simulink model "LabB_PIDOverRobot"  (R2019b)
settings: Solver=FixedStepDiscrete  StartTime=0.0  StopTime=inf  FixedStep=fSamplingPeriod  RelTol=1e-3  EnableMultiTasking=on
values from neighbouring files (symbols this model uses):
  fGyroBias = -315    [GyroBias.mat]
  fGyroConversionFactor = -1/131    (= -0.00763358778626)    [LabB_ObserverAndControllerOverRobot_Parameters.m]    (also in LabB_PIDOverRobot_Parameters.m; LabC_Servo.m; LabC_observer.m; LoadRobotParameters.m = 0.00762939453125)
  fSamplingPeriod = 0.005    [LabB_ControllerOverSimulator_Discrete_Parameters.m]    (also in LabB_ObserverAndControllerOverRobot_Parameters.m = 0.01; LabB_ObserverAndControllerOverSimulator_Discrete_Parameters.m = 0.01; LabB_ObserverOverSimulator_Discrete_Parameters.m = 0.01; LabB_PIDOverRobot_Parameters.m)
  fWheelRadius = 0.0216    [LabB_ObserverAndControllerOverRobot_Parameters.m]    (also in LabB_PIDOverRobot_Parameters.m; LabC_Servo.m; LabC_observer.m; LoadRobotParameters.m)
  iNumberOfEncoderSteps = 720    [LabB_ObserverAndControllerOverRobot_Parameters.m]    (also in LabB_PIDOverRobot_Parameters.m; LabC_Servo.m; LabC_observer.m; LoadRobotParameters.m)
  kD = -0.0554    [LabB_ObserverAndControllerOverRobot_Parameters.m]    (also in LabB_ObserverAndControllerOverSimulator_Discrete_Parameters.m; LabB_ObserverOverSimulator_Continuous_Parameters.m = -0.0553889349754; LabB_ObserverOverSimulator_Discrete_Parameters.m = -0.0553889349754; LabB_PIDOverRobot_Parameters.m = -0.05538361401)
  kI = -263.4728    [LabB_ObserverAndControllerOverRobot_Parameters.m]    (also in LabB_ObserverAndControllerOverSimulator_Discrete_Parameters.m; LabB_ObserverOverSimulator_Continuous_Parameters.m = -263.472756557; LabB_ObserverOverSimulator_Discrete_Parameters.m = -263.472756557; LabB_PIDOverRobot_Parameters.m = -263.540867)
  kP = -47.0274    [LabB_ObserverAndControllerOverRobot_Parameters.m]    (also in LabB_ObserverAndControllerOverSimulator_Discrete_Parameters.m; LabB_ObserverOverSimulator_Continuous_Parameters.m = -47.0274213515; LabB_ObserverOverSimulator_Discrete_Parameters.m = -47.0274213515; LabB_PIDOverRobot_Parameters.m = -47.0230144)
undefined symbols (not defined in the file or in its folder): DiscIntNeverNeededParam
libraries: MinSegLibrary_M2V3 x3, simulink x1
settings Model: FPTRunName=FPA_Reference  ExtModeTrigDuration=2  Creator=Alec  LastModifiedBy=jlosi
settings DataIOCC: SaveFormat=Array  SaveOutput=off  SignalLogging=off  DSMLogging=off  SaveTime=off  ReturnWorkspaceOutputs=off
settings OptimizationCC: PassReuseOutputArgsAs=Individual arguments  ExpressionDepthLimit=2147483647  MaxStackSize=64  EfficientTunableParamExpr=on
settings DebuggingCC: UnderspecifiedInitializationDetection=Classic  MergeDetectMultiDrivingBlocksExec=none  ParameterTunabilityLossMsg=error  StateNameClashWarn=warning  SFUnexpectedBacktrackingDiag=warning  SFNoUnconditionalDefaultTransitionDiag=warning  SFExecutionAtInitializationDiag=none  ArithmeticOperatorsInVariantConditions=warning
settings HardwareCC: ProdBitPerInt=16  ProdBitPerPointer=16  ProdBitPerSizeT=16  ProdBitPerPtrDiffT=16  ProdLargestAtomicFloat=None  ProdWordSize=8  ProdHWDeviceType=Atmel->AVR
settings ModelReferenceCC: PropagateSignalLabelsOutOfModel=off
settings SFSimCC: SimUseLocalCustomCode=off  MATLABDynamicMemAlloc=off  CustomCodeUndefinedFunction=UseInterfaceOnly
settings RTWCC: SystemTargetFile=ert.tlc  HardwareBoard=Arduino Mega 2560  TLCOptions=-aInlineSetEventsForThisBaseRateFcn=TLC_FALSE -aSuppressMultiTaskScheduler=TLC_FALSE -aRateBasedStepFcn=1  TemplateMakefile=ert_default_tmf  GenerateReport=on  RTWVerbose=off  RTWUseLocalCustomCode=off  Toolchain=Arduino AVR  BuildConfiguration=Faster Runs  IncludeHyperlinkInReport=on  LaunchReport=on  GenerateTraceInfo=on  GenerateTraceReport=on  GenerateTraceReportSl=on  GenerateTraceReportSf=on  GenerateTraceReportEml=on
settings CodeAppCC: ForceParamTrailComments=on  IgnoreCustomStorageClasses=off  OperatorAnnotations=on  SimulinkDataObjDesc=on  SFDataObjDesc=on  MATLABFcnDesc=on  CustomSymbolStrType=$N$R$M  InsertBlockDesc=on  StateflowObjectComments=on  MATLABSourceComments=on  InternalIdentifier=Classic
settings ERTTargetCC: SupportContinuousTime=on  SupportVariableSizeSignals=on
settings ConfigComp: CovMetricSettings=dw  CovHtmlReporting=on  CovSaveCumulativeToWorkspaceVar=on  CovSaveSingleToWorkspaceVar=on  CovExternalEMLEnable=off

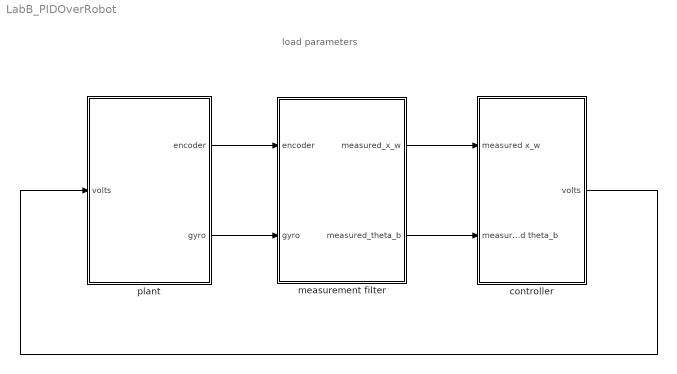
== system LabB_PIDOverRobot ==
  note: load parameters
  controller : Subsystem
  measurement filter : Subsystem
  plant : Subsystem
  wires:
  controller/1(volts) -> plant/1(volts)
  plant/2(gyro) -> measurement filter/2(gyro)
  measurement filter/2(measured_theta_b) -> controller/2("measured theta_b ")
  measurement filter/1(measured_x_w) -> controller/1(measured x_w)
  plant/1(encoder) -> measurement filter/1(encoder)

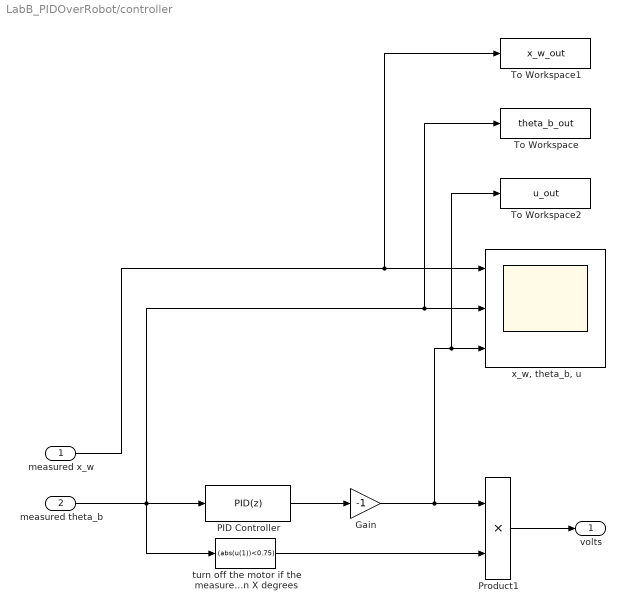
== system LabB_PIDOverRobot/controller ==
  measured x_w : Inport
  "measured theta_b " : Inport  Port=2
  Gain : Gain  Gain=-1
  PID Controller : simulink/Continuous/PID Controller  Controller=PID  Form=Parallel  TimeDomain=Discrete-time  SampleTime=fSamplingPeriod  IntegratorMethod=Forward Euler  FilterMethod=Forward Euler  ControllerParametersSource=internal  P=-kP  I=-kI  D=-kD  UseFilter=on  N=100  TunerSelectOption=Transfer Function Based (PID Tuner App)  InitialConditionSource=internal  InitialConditionForIntegrator=0  InitialConditionForFilter=0  DifferentiatorICPrevScaledInput=0  ExternalReset=none  TrackingMode=off  Kt=1  LimitOutput=on  UpperSaturationLimit=6  LowerSaturationLimit=-6  LinearizeAsGain=on  AntiWindupMode=back-calculation  Kb=1  POutMin=[]  POutMax=[]  IOutMin=[]  IOutMax=[]  DOutMin=[]  DOutMax=[]  NOutMin=[]  NOutMax=[]  SumOutMin=[]  SumOutMax=[]  SaturationOutMin=[]  SaturationOutMax=[]  PParamMin=[]  PParamMax=[]  IParamMin=[]  IParamMax=[]  DParamMin=[]  DParamMax=[]  NParamMin=[]  NParamMax=[]  KbParamMin=[]  KbParamMax=[]  KtParamMin=[]  KtParamMax=[]  KbOutMin=[]  KbOutMax=[]  KtOutMin=[]  KtOutMax=[]  IntegratorOutMin=[]  IntegratorOutMax=[]  FilterOutMin=[]  FilterOutMax=[]  SumI1OutMin=[]  SumI1OutMax=[]  SumI2OutMin=[]  SumI2OutMax=[]  SumI3OutMin=[]  SumI3OutMax=[]  SumI4OutMin=[]  SumI4OutMax=[]  SumDOutMin=[]  SumDOutMax=[]  DifferentiatorOutMin=[]  DifferentiatorOutMax=[]  FilterDiffOutCoefMin=[]  FilterDiffOutCoefMax=[]  ReciprocalOutMin=[]  ReciprocalOutMax=[]  SumDenOutMin=[]  SumDenOutMax=[]  SumNumOutMin=[]  SumNumOutMax=[]  DivideOutMin=[]  DivideOutMax=[]  IntegratorContinuousStateAttributes=''  IntegratorStateMustResolveToSignalObject=off  IntegratorRTWStateStorageClass=Auto  FilterContinuousStateAttributes=''  FilterStateMustResolveToSignalObject=off  FilterRTWStateStorageClass=Auto  ParallelPVariant=InternalParameters  IdealPVariant=Disabled  IVariant=InternalParameters  DVariant=InternalParameters  IntegratorVariant=Discrete  SatVariant=Enabled  AWVariant=BackCalculation  PCopyVariant=Disabled  TRVariant=Disabled  FdbkBlocksVariant=Forward  IdealPFdbkVariant=Disabled  SatFdbkVariant=Disabled  DerivativeFilterVariant=ForwardEulerFilter  NVariant=InternalParameters  NCopyVariant=Disabled  FilterICVariant=InternalICsFilter  IntegratorICVariant=InternalICs  ExternalResetVariant=Disabled  TRSumVariant=Passthrough  SumFdbkVariant=Disabled  SumVariant=Sum_PID
  Product1 : Product  RndMeth=Zero
  To Workspace : ToWorkspace  VariableName=theta_b_out  SaveFormat=Structure With Time  SampleTime=-1
  To Workspace1 : ToWorkspace  VariableName=x_w_out  SaveFormat=Structure With Time  SampleTime=-1
  To Workspace2 : ToWorkspace  VariableName=u_out  SaveFormat=Structure With Time  SampleTime=-1
  turn off the motor if the measured angle is greater than X degrees : Fcn  Expr=(abs(u(1))<0.75)
  "x_w, theta_b, u" : Scope  NumInputPorts=3
  volts : Outport  VectorParamsAs1DForOutWhenUnconnected=off
  wires:
  "measured theta_b "/1 -> To Workspace/1, "x_w, theta_b, u"/2, turn off the motor if the measured angle is greater than X degrees/1, PID Controller/1
  Product1/1 -> volts/1
  turn off the motor if the measured angle is greater than X degrees/1 -> Product1/2
  PID Controller/1 -> Gain/1
  measured x_w/1 -> To Workspace1/1, "x_w, theta_b, u"/1
  Gain/1 -> To Workspace2/1, "x_w, theta_b, u"/3, Product1/1

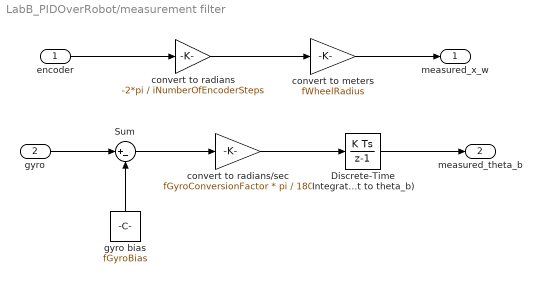
== system LabB_PIDOverRobot/measurement filter ==
  encoder : Inport
  gyro : Inport  Port=2
  Discrete-Time Integrator (convert from theta_b_dot to theta_b) : DiscreteIntegrator  SampleTime=fSamplingPeriod  OutDataTypeStr=Inherit: Inherit via back propagation  ICPrevOutput=DiscIntNeverNeededParam  ICPrevScaledInput=DiscIntNeverNeededParam
  Sum : Sum  Inputs=|+-
  convert to radians/sec : Gain  Gain=fGyroConversionFactor * pi / 180  OutDataTypeStr=Inherit: Same as input
  convert to radians : Gain  Gain=-2*pi / iNumberOfEncoderSteps  OutDataTypeStr=Inherit: Same as input
  convert to meters : Gain  Gain=fWheelRadius  OutDataTypeStr=Inherit: Same as input
  gyro bias : Constant  Value=fGyroBias  OutDataTypeStr=single
  measured_x_w : Outport  VectorParamsAs1DForOutWhenUnconnected=off
  measured_theta_b : Outport  Port=2  VectorParamsAs1DForOutWhenUnconnected=off
  wires:
  convert to radians/sec/1 -> Discrete-Time Integrator (convert from theta_b_dot to theta_b)/1
  gyro/1 -> Sum/1
  Sum/1 -> convert to radians/sec/1
  convert to radians/1 -> convert to meters/1
  encoder/1 -> convert to radians/1
  Discrete-Time Integrator (convert from theta_b_dot to theta_b)/1 -> measured_theta_b/1
  gyro bias/1 -> Sum/2
  convert to meters/1 -> measured_x_w/1

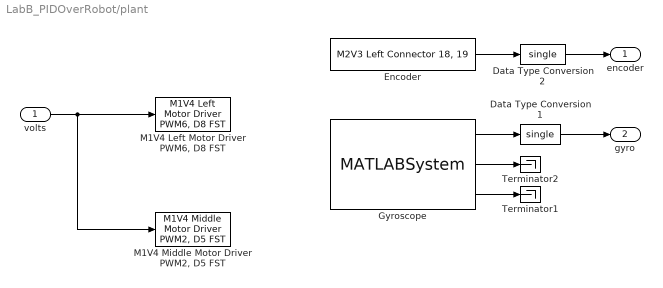
== system LabB_PIDOverRobot/plant ==
  volts : Inport
  Data Type Conversion1 : DataTypeConversion  OutDataTypeStr=single
  Data Type Conversion2 : DataTypeConversion  OutDataTypeStr=single
  Encoder : MinSegLibrary_M2V3/M2V3 Left Connector 18, 19  Encoder=1  PinA=19  PinB=18
      settings: SourceProductName=Rensselaer Arduino Support Package
  Gyroscope : MATLABSystem  System=soMPU6050Gyro  DLPFmode=0
      mask Type: soMPU6050Gyro
      mask Display:
      | disp('soMPU6050Gyro');
      | port_label('output',1,'xvel');
      | port_label('output',2,'yvel');
      | port_label('output',3,'zvel');
  "M1V4 Left Motor Driver PWM6, D8 FST" : MinSegLibrary_M2V3/M1V4 Left Motor Driver PWM6, D8 FST  Vsupply=7.2
      settings: SourceProductName=Rensselaer Arduino Support Package
  "M1V4 Middle Motor Driver PWM2, D5 FST" : MinSegLibrary_M2V3/M1V4 Middle Motor Driver PWM2, D5 FST  Vsupply=7.2
      settings: SourceProductName=Rensselaer Arduino Support Package
  Terminator1 : Terminator
  Terminator2 : Terminator
  encoder : Outport  VectorParamsAs1DForOutWhenUnconnected=off
  gyro : Outport  Port=2  VectorParamsAs1DForOutWhenUnconnected=off
  wires:
  Gyroscope/1 -> Data Type Conversion1/1
  Data Type Conversion1/1 -> gyro/1
  Encoder/1 -> Data Type Conversion2/1
  Data Type Conversion2/1 -> encoder/1
  Gyroscope/3 -> Terminator1/1
  Gyroscope/2 -> Terminator2/1
  volts/1 -> "M1V4 Middle Motor Driver PWM2, D5 FST"/1, "M1V4 Left Motor Driver PWM6, D8 FST"/1
